simulink subsystem "thermal_emitters"  (R2024b)
settings: Solver=VariableStepAuto  StartTime=0.0  StopTime=10.0  RelTol=1e-3
model mask{m_min=0.4, n_radiators=12, n_tubes=2, D=0.02, L=3, U=50, T_air=20}
  mask prompts: m_min "m_min: non-zero velocity mass flow (for dt=10s, see function doc) [kg/s]"; n_radiators "Number of radiators"; n_tubes "Number of tubes per radiator"; D "Diameter of each tube [m]"; L "Length of each tube [m]"; U "Overall heat exchange coefficient [W/(m2.K)]"; T_air "Surrounding air temperature [°C]"
settings Model: Creator=nerotb  LastModifiedBy=nerotb

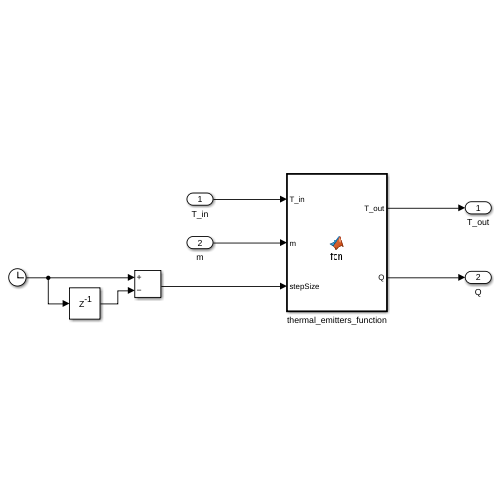
[thumbnail: Simulink's stored preview of the top-level diagram]
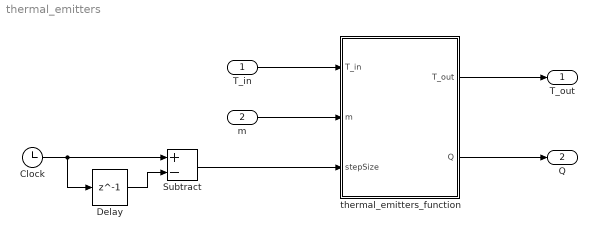
== system thermal_emitters ==
  T_in : Inport
  m : Inport  Port=2
  Clock : Clock
  Delay : Delay  DelayLength=1  InputProcessing=Columns as channels (frame based)
  Subtract : Sum  Inputs=+-
  thermal_emitters_function : MATLAB Function  TreatAsAtomicUnit=on
  T_out : Outport
  Q : Outport  Port=2
  wires:
  T_in/1 -> thermal_emitters_function/1(T_in)
  m/1 -> thermal_emitters_function/2(m)
  thermal_emitters_function/1(T_out) -> T_out/1
  thermal_emitters_function/2(Q) -> Q/1
  Subtract/1 -> thermal_emitters_function/3(stepSize)
  Clock/1 -> Delay/1, Subtract/1
  Delay/1 -> Subtract/2

== matlab function thermal_emitters/thermal_emitters_function ==
  data: T_in input size=1; m input size=1; T_out output size=1; Q output size=1; U parameter; D parameter; T_air parameter; stepSize input; L parameter; n_radiators parameter; n_tubes parameter; m_min parameter
function [T_out, Q] = fcn(T_in, m, U, D, T_air, stepSize, L, n_radiators, n_tubes, m_min)
%% Summary
% This function models the thermal exchange that occurs in several
% identical space heating thermal emitters (=radiators).
%
% See the "About m_min" before use.

%% Model
% There are `n_radiators` radiators. Each of them is a parallel assembly of
% `n_tubes` cylindrical tubes. Thus each tube is filled with water at mass
% flow m / (n_radiators * n_tubes).
% Thermal exchange occurs between these tubes and indoor air at temperature
% `T_in`.
% The model of each tube is very similar to the model of thermal pipes.
% The tube is discretized in a 1D mesh. 

%% About m_min
% The size of the mesh is determined by `m_min`. 
% `m_min` is the minimum mass flow `m` for water to move in each tube.
%
% - if m > m_min: the temperatures distribution varies due to both 
% nonzero velocity of the flow and thermal exchange with the air (space heating)
% - if m < m_min: the flow is motionless in the tubes, 
% but thermal exchange with the air still occurs
%
% A low `m_min` creates a fine mesh, coming with higher algorithmic
% complexity.
%
% m_min is defined for a macro time step of dt_=10 seconds. 
%   If you use a larger time step dt and want to use a m_min value m_min(@dt), 
%   then provide m_min as:
%      m_min = m_min(@dt_) = C * (dt / dt_) * m_min(@dt) 
%                          = C * (dt / 10)  * m_min(@dt)
% For some discreet effects reasons in the meshing definition, 
% it is recommended to apply a safety coefficient C = 0.6.

%% About the macro time step
% For the same reasons as the storage_TC component, 
% macro time step must be constant during the simulation.

%% Parameters
% U: overall thermal exchange coefficient [W/(m2.K)]
% n_radiators: number of radiators [-]
% n_tubes: number of tubes per radiator [-]
% D: diameter of each tube [m]
% L: length of each tube [m]
% T_air: indoor air temperature [°C]
% m_min: minimum mass flow for the water not to stagnate within each tube [kg/s]

%% Variables
% Q: exchanged thermal power [W]
% m: total mass flow circulating in all radiators [kg/s]
% T_in: entering temperature of the flow [°C]
% T_out: exiting temperature of the flow [°C]
%       computed as the temporal average over the ode solving duration
%       (=macro time step)
%       of the temperature of the last node 
%       (i.e. end of the tube, where water exits)

%% Hypothesis
% - The thermal exchange occurs without any change in air temperature at the vicinity of the radiators.
% - Cp is constant

%% Initialization
% At simulation start, the temperature profile along each tube is uniform
% with value T_air.

%% Algorithmic complexity:
% There are:
%   - n variables (temperature distribution along the tube, all tubes are the same)
%   - n equations 
%
% The smaller m_min the larger n.


persistent T
persistent A
persistent rho
persistent timeIdx    % index of macro time step, starts at 1
persistent oldStepSize
persistent n_dx       % number of meshing nodes
persistent dx         % length of a node [m]
persistent tau

if isempty(tau)
    Cp = 4180;
    rho = 1000;
    A = pi * D * D / 4;
    oldStepSize = -1;
    timeIdx = 1;
    tau = rho*D*Cp / (4*U);
    % meshing of tubes:
    % the length of a node (dx) is the distance the water flow covers at the velocity V_min during a duration dt_=10s
    % --> dt_ is independant from the real macro time step because this time step is unknown at first call of the function (see oldStepSize)
    % --> if water velocity is V < V_min, it is set to 0 (equivalent to m=0)
    
    dt_ = 10;
    V_min_tube = (m_min / (rho * A)) / (n_tubes * n_radiators);
    dx_ = V_min_tube * dt_;
    n_dx = floor(L / dx_);    
    n_dx = max(n_dx, 1);
    dx = L / n_dx;           

    T = ones(1, n_dx) * T_air;
    fprintf("Thermal emitters: meshing created %d nodes.\n", int32(n_dx));

else
    timeIdx = timeIdx + 1;
end


if timeIdx == 1
    % initial stepSize value (0) is wrong, 
    % it is replaced by a reasonnable value
    stepSize = 30;
elseif timeIdx == 2
    oldStepSize = stepSize;
else
    assert(abs(oldStepSize - stepSize) < 1e-3) % could be replaced by a call to `isapprox` 
                                               % but this function is not compatible with C-code generation
end


dt = stepSize;    

% m_min is redefined given real macro time step
V_min_tube = dx / dt;
m_min = V_min_tube * n_tubes * n_radiators * rho * A;
if timeIdx == 3
    fprintf("Thermal emitters: m_min=%1.2e kg/s (for dt=%1.1fs).\n", m_min, dt);
end

if m < 0
    fprintf("Thermal emitters: mass flow m=%1.2e kg/s < 0, it is replaced by zero.\n", m);
    m = 0;
elseif (0 < m) && (m <= m_min)
    fprintf("Thermal emitters: mass flow m=%1.2e kg/s too small for the meshing (m_min value (for dt=%1.1fs): %1.2e kg/s), " + ...
        "it is replaced by zero.\n", m, dt, m_min);
    m = 0;
end

V = m / (rho * A * n_tubes * n_radiators);      % velocity in each tube [m/s]
t0 = 0;
tf = dt;



function out=ODE(t, y, V, T_in)

    % y = [T1, ... , Tn]        n values
    out = zeros(n_dx, 1);

    % node 1
    out(1) =     - (V/dx + 1 / tau) * y(1) + 1 / tau * T_air + V * T_in / dx;

    % node i: 2 to n
    for i=2:n_dx
        out(i) = - (V/dx + 1 / tau) * y(i) + 1 / tau * T_air + V * y(i-1) / dx;
    end

end


tspan = t0:tf;
options = odeset('RelTol',1e-3, 'AbsTol', 1e-3);

y0 = T;
[~,y] = ode23(@(t, y) ODE(t, y, V, T_in), tspan, y0, options); 
Q = n_radiators * n_tubes * U * pi * D * L * (mean(y, "all") - T_air);
T_out = mean(y(:, end));
T = y(end, :);


end
